simulink model "project_2_hw"  (R2020a)
settings: Solver=VariableStepAuto  StartTime=0.0  StopTime=10.0  RelTol=1e-3
libraries: simulink x1
settings Model: Creator=Matt  LastModifiedBy=Matt
settings DataIOCC: ReturnWorkspaceOutputs=off

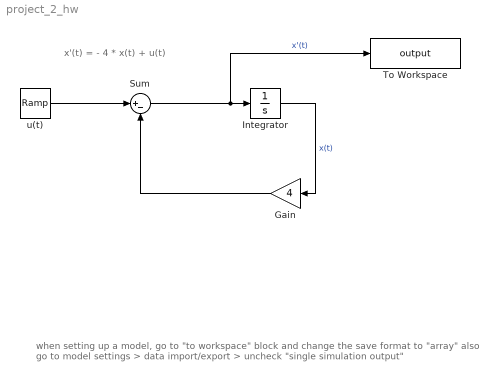
== system project_2_hw ==
  note: x'(t) = - 4 * x(t) + u(t)
  note: when setting up a model, go to "to workspace" block and change the save format to "array"
      | also go to model settings > data import/export > uncheck "single simulation output"
  Gain : Gain  Gain=4
  Integrator : Integrator
  Sum : Sum  Inputs=|+-
  To Workspace : ToWorkspace  VariableName=output  SampleTime=-1
  u(t) : simulink/Sources/Ramp  slope=1  start=0  InitialOutput=0
  wires:
  u(t)/1 -> Sum/1
  Gain/1 -> Sum/2
  Sum/1 -> To Workspace/1, Integrator/1  "x'(t)"
  Integrator/1 -> Gain/1  "x(t)"
